simulink model "dc2_megfigyelo_afa"  (R2013a)
settings: Solver=VariableStepDiscrete  StartTime=0.0  StopTime=200  RelTol=1e-3
undefined symbols (not defined in the file or in its folder): j
settings Model: Creator=balazs.varga  LastModifiedBy=balazs.varga

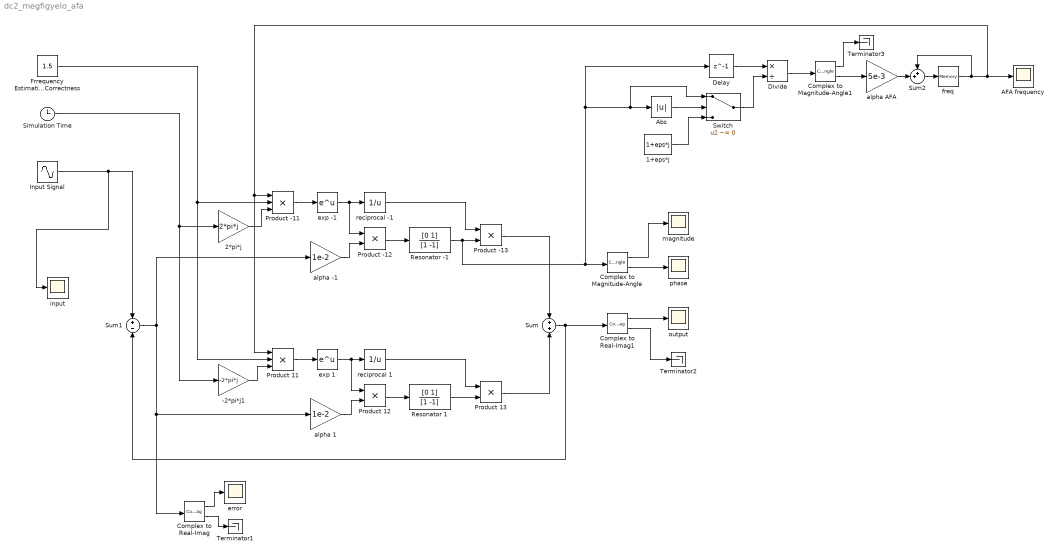
== system dc2_megfigyelo_afa ==
  -2*pi*j1 : Gain  Gain=-2*pi*j  SampleTime=1e-3
  1+eps*j : Constant  Value=1+eps*j
  2*pi*j : Gain  Gain=2*pi*j  SampleTime=1e-3
  AFA frequency : Scope
      settings: YMin=0.7  YMax=1  SaveName=ScopeData5
  Abs : Abs
  Complex to Magnitude-Angle : ComplexToMagnitudeAngle  SampleTime=1e-3
  Complex to Magnitude-Angle1 : ComplexToMagnitudeAngle  SampleTime=1e-3
  Complex to Real-Imag : ComplexToRealImag  SampleTime=1e-3
  Complex to Real-Imag1 : ComplexToRealImag  SampleTime=1e-3
  Delay : Delay  DelayLength=1  InitialCondition=0  SampleTime=1e-3
  Divide : Product  Inputs=*/  SampleTime=1e-3
  Frrequency Estimation Correctness : Constant  Value=1.5
  Input Signal : Sin  Frequency=2*pi  Phase=1  SampleTime=0
  Product -11 : Product  Inputs=3  SampleTime=1e-3
  Product -12 : Product  SampleTime=1e-3
  Product -13 : Product  SampleTime=1e-3
  Product 11 : Product  Inputs=3  SampleTime=1e-3
  Product 12 : Product  SampleTime=1e-3
  Product 13 : Product  SampleTime=1e-3
  Resonator -1 : DiscreteFilter  Numerator=[0 1]  Denominator=[1 -1]  SampleTime=1e-3
  Resonator 1 : DiscreteFilter  Numerator=[0 1]  Denominator=[1 -1]  SampleTime=1e-3
  Simulation Time : Clock
  Sum : Sum  Inputs=+|+  SampleTime=1e-3
  Sum1 : Sum  Inputs=+|-  SampleTime=1e-3
  Sum2 : Sum  Inputs=++|  SampleTime=1e-3
  Switch : Switch  Criteria=u2 ~= 0  SampleTime=1e-3
  Terminator1 : Terminator
  Terminator2 : Terminator
  Terminator3 : Terminator
  alpha -1 : Gain  Gain=1e-2  SampleTime=1e-3
  alpha 1 : Gain  Gain=1e-2  SampleTime=1e-3
  alpha AFA : Gain  Gain=5e-3  SampleTime=1e-3
  error : Scope
      settings: YMin=-0.4  YMax=1.3
  exp -1 : Math  SampleTime=1e-3  SaturateOnIntegerOverflow=on
  exp 1 : Math  SampleTime=1e-3  SaturateOnIntegerOverflow=on
  freq : Memory  X0=1  InheritSampleTime=on
  input : Scope
      settings: SaveName=ScopeData2
  magnitude : Scope
      settings: YMin=0  YMax=0.7  SaveName=ScopeData3
  output : Scope
  phase : Scope
      settings: SaveName=ScopeData4
  reciprocal -1 : Math  Operator=reciprocal  SampleTime=1e-3  SaturateOnIntegerOverflow=on
  reciprocal 1 : Math  Operator=reciprocal  SampleTime=1e-3  SaturateOnIntegerOverflow=on
  wires:
  Product -12/1 -> Resonator -1/1
  Product 12/1 -> Resonator 1/1
  Product -11/1 -> exp -1/1
  Product 11/1 -> exp 1/1
  exp -1/1 -> reciprocal -1/1, Product -12/1
  reciprocal -1/1 -> Product -13/1
  exp 1/1 -> reciprocal 1/1, Product 12/1
  Resonator 1/1 -> Product 13/2
  reciprocal 1/1 -> Product 13/1
  Product -13/1 -> Sum/1
  Product 13/1 -> Sum/2
  Sum/1 -> Complex to Real-Imag1/1, Sum1/2
  Sum1/1 -> alpha -1/1, Complex to Real-Imag/1, alpha 1/1
  Complex to Real-Imag/1 -> error/1
  Complex to Real-Imag1/1 -> output/1
  Input Signal/1 -> input/1, Sum1/1
  Complex to Magnitude-Angle/1 -> magnitude/1
  Complex to Magnitude-Angle/2 -> phase/1
  Frrequency Estimation Correctness/1 -> Product 11/2, Product -11/2
  Resonator -1/1 -> Switch/1, Abs/1, Delay/1, Complex to Magnitude-Angle/1, Product -13/2
  Simulation Time/1 -> -2*pi*j1/1, 2*pi*j/1
  Divide/1 -> Complex to Magnitude-Angle1/1
  Abs/1 -> Switch/2
  Complex to Magnitude-Angle1/2 -> alpha AFA/1
  1+eps*j/1 -> Switch/3
  Sum2/1 -> freq/1
  alpha AFA/1 -> Sum2/2
  freq/1 -> Product -11/1, Product 11/1, AFA frequency/1, Sum2/1
  Switch/1 -> Divide/2
  Delay/1 -> Divide/1
  Complex to Real-Imag/2 -> Terminator1/1
  Complex to Real-Imag1/2 -> Terminator2/1
  Complex to Magnitude-Angle1/1 -> Terminator3/1
  2*pi*j/1 -> Product -11/3
  -2*pi*j1/1 -> Product 11/3
  alpha 1/1 -> Product 12/2
  alpha -1/1 -> Product -12/2
